simulink model "youbot_pd_control_ros"  (R2018b)
settings: Solver=FixedStepAuto  StartTime=0.0  StopTime=inf  RelTol=1e-3
libraries: robotlib x3
settings Model: Creator=kika  LastModifiedBy=kika

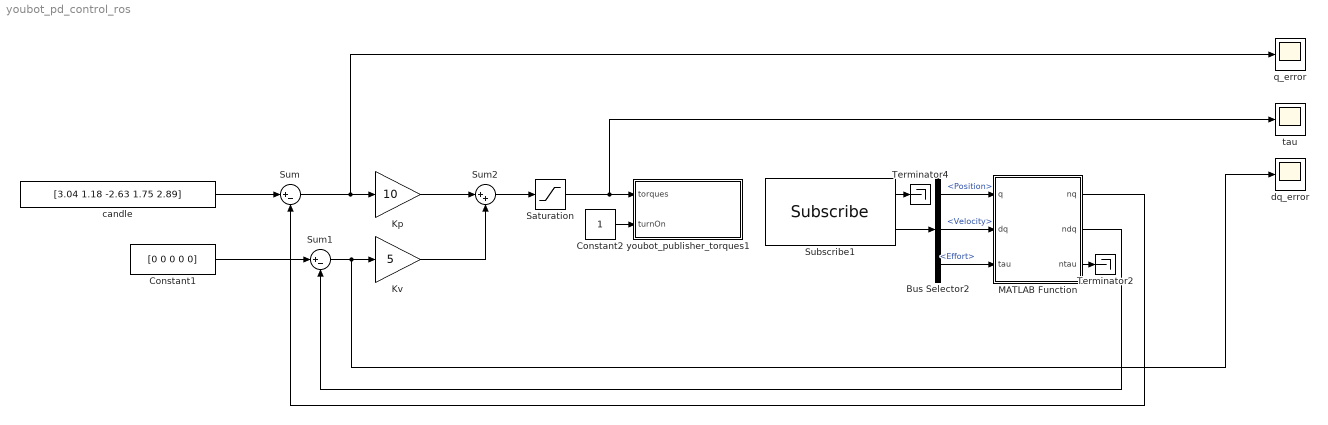
== system youbot_pd_control_ros ==
  Bus Selector2 : BusSelector  OutputSignals=Position,Velocity,Effort
  Constant1 : Constant  Value=[0 0 0 0 0]
  Constant2 : Constant
  Kp : Gain  Gain=10
  Kv : Gain  Gain=5
  MATLAB Function : MATLAB Function  TreatAsAtomicUnit=on
  Saturation : Saturate  UpperLimit=8  LowerLimit=-8
  Subscribe1 : robotlib/Subscribe  topicSource=Select from ROS network  topic=/joint_states  messageType=sensor_msgs/JointState  sampleTime=-1  messageQueueLength=1
      settings: SourceProductBaseCode=RO
  Sum : Sum  Inputs=|+-
  Sum1 : Sum  Inputs=|+-
  Sum2 : Sum  Inputs=|++
  Terminator2 : Terminator
  Terminator4 : Terminator
  candle : Constant  Value=[3.04 1.18 -2.63 1.75 2.89]
  dq_error : Scope
  q_error : Scope
  tau : Scope
  youbot_publisher_torques1 : Subsystem
  wires:
  candle/1 -> Sum/1
  Constant1/1 -> Sum1/1
  Sum/1 -> Kp/1, q_error/1
  Kp/1 -> Sum2/1
  Kv/1 -> Sum2/2
  Sum2/1 -> Saturation/1
  MATLAB Function/3(ntau) -> Terminator2/1
  MATLAB Function/2(ndq) -> Sum1/2
  Saturation/1 -> tau/1, youbot_publisher_torques1/1(torques)
  MATLAB Function/1(nq) -> Sum/2
  Subscribe1/2 -> Bus Selector2/1
  Subscribe1/1 -> Terminator4/1
  Constant2/1 -> youbot_publisher_torques1/2(turnOn)
  Bus Selector2/3 -> MATLAB Function/3(tau)  "<Effort>"
  Bus Selector2/2 -> MATLAB Function/2(dq)  "<Velocity>"
  Bus Selector2/1 -> MATLAB Function/1(q)  "<Position>"
  Sum1/1 -> Kv/1, dq_error/1

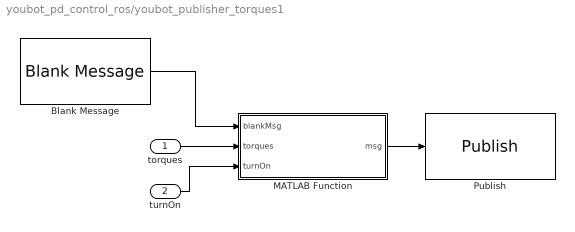
== system youbot_pd_control_ros/youbot_publisher_torques1 ==
  torques : Inport
  turnOn : Inport  Port=2
  Blank Message : robotlib/Blank Message  messageClass=Message  entityType=brics_actuator/JointTorques  messageType=brics_actuator/JointTorques  SampleTime=inf
      settings: SourceProductBaseCode=RO
  MATLAB Function : MATLAB Function  TreatAsAtomicUnit=on
  Publish : robotlib/Publish  topicSource=Select from ROS network  topic=/arm_1/arm_controller/torques_command  messageType=brics_actuator/JointTorques  messageQueueLength=1
      settings: SourceProductBaseCode=RO
  wires:
  MATLAB Function/1(msg) -> Publish/1
  torques/1 -> MATLAB Function/2(torques)
  Blank Message/1 -> MATLAB Function/1(blankMsg)
  turnOn/1 -> MATLAB Function/3(turnOn)

== matlab function youbot_pd_control_ros/MATLAB Function ==
  data: q input; nq output; dq input; tau input; ndq output; ntau output
function [nq, ndq, ntau] = ros_to_matlab(q, dq, tau)

nq = q(1:5);
ndq = dq(1:5);
ntau = tau(1:5); % need minus??

== matlab function youbot_pd_control_ros/youbot_publisher_torques1/MATLAB Function ==
  settings: updateMethod=DISCRETE
  data: blankMsg input; msg output Bus: SL_Bus_youbot_pd_control_ROS_brics_actuator_JointTorques; torques input; turnOn input
function msg = setTorque(blankMsg, torques, turnOn)
    persistent Sec
    if isempty(Sec)
        Sec = 0;
    end
    
    n = 5;
    uri = 'arm_joint_';
    unit = 'm^2 kg s^-2 rad^-1';

    blankMsg.Torques_SL_Info.CurrentLength = uint32(n);

    for i = 1:n
        %bmsg.Torques(i).TimeStamp.Sec = Sec;   

        strLength = length(uri) + 1;    % plus index of joint
        blankMsg.Torques(i).JointUri(1:strLength) = [uint8(uri), uint8(i + 48)]; % shift in ascii table for number '0'
        blankMsg.Torques(i).JointUri_SL_Info.CurrentLength = uint32(strLength);

        strLength = length(unit);
        blankMsg.Torques(i).Unit(1:strLength) = uint8(unit);
        blankMsg.Torques(i).Unit_SL_Info.CurrentLength = uint32(strLength);

        if turnOn
            blankMsg.Torques(i).Value = torques(i);
        else
            blankMsg.Torques(i).Value = 0;
        end

    end
    Sec = Sec + 1;
    msg = blankMsg;    
end
